simulink model "SPI_controller"  (R2014b)
settings: Solver=FixedStepDiscrete  StartTime=0.0  StopTime=100000  FixedStep=1  RelTol=1e-3
model workspace (MAT data in the model file):
  message_length = Simulink.Parameter
  message_length.Value = 16
  message_length.DataType = 'uint16'
  clk_freq = Simulink.Parameter
  clk_freq.Value = 1000000
  clk_freq.DataType = 'uint32'
  cs_to_clk_edge = Simulink.Parameter
  cs_to_clk_edge.Value = 10
  cs_to_clk_edge.DataType = 'uint16'
  stall_time = Simulink.Parameter
  stall_time.Value = 4
  stall_time.DataType = 'uint16'
undefined symbols (not defined in the file): read_table
libraries: simulink x9, hdlsllib x1
settings Model: FPTRunName=FPA_Reference  Creator=bsoheili  LastModifiedBy=dlwalter
settings DataIOCC: SaveOutput=off  SaveTime=off
settings OptimizationCC: BlockReduction=off  ConditionallyExecuteInputs=off  InlineParams=on  UseDivisionForNetSlopeComputation=UseDivisionForReciprocalsOfIntegersOnly  UseFloatMulNetSlope=on  InlineInvariantSignals=on  EnhancedBackFolding=on  EfficientFloat2IntCast=on  OptimizeModelRefInitCode=on  LifeSpan=1  SimCompilerOptimization=off
settings DebuggingCC: SignalRangeChecking=warning  AlgebraicLoopMsg=error  InheritedTsInSrcMsg=none  ParameterDowncastMsg=warning  ParameterOverflowMsg=warning  FrameProcessingCompatibilityMsg=error  StrictBusMsg=ErrorOnBusTreatedAsVector  NonBusSignalsTreatedAsBus=error
settings HardwareCC: ProdHWDeviceType=ASIC/FPGA->ASIC/FPGA  ProdEqTarget=off
settings RTWCC: SystemTargetFile=ert.tlc  TemplateMakefile=ert_default_tmf  Description=Embedded Coder  GenerateReport=on  IncludeHyperlinkInReport=on  LaunchReport=on  GenerateTraceInfo=on  GenerateTraceReport=on  GenerateTraceReportSl=on  GenerateTraceReportSf=on  GenerateTraceReportEml=on  GenerateCodeMetricsReport=on  RTWCompilerOptimization=off
settings CodeAppCC: IgnoreCustomStorageClasses=off
settings ERTTargetCC: GenerateSampleERTMain=on  CombineSignalStateStructs=on  SuppressErrorStatus=on  InlinedParameterPlacement=NonHierarchical  ERTCustomFileTemplate=example_file_process.tlc

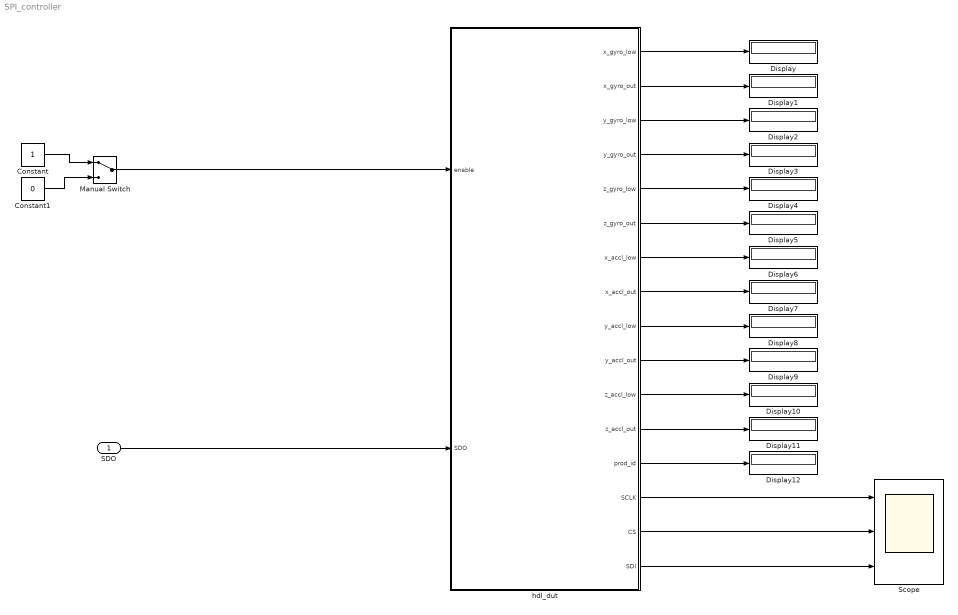
== system SPI_controller ==
  SDO : Inport
  Constant : Constant  OutDataTypeStr=boolean  SampleTime=-1
  Constant1 : Constant  Value=0  OutDataTypeStr=boolean  SampleTime=-1
  Display{,1..12} (13 alike) : Display
  Manual Switch : ManualSwitch
  Scope : Scope  NumInputPorts=3
      settings: TimeRange=3000  YMin=-5~-5~-5  YMax=5~5~5
  hdl_dut : Subsystem  TreatAsAtomicUnit=on  MinMaxOverflowLogging=MinMaxAndOverflow
  wires:
  Manual Switch/1 -> hdl_dut/1(enable)
  SDO/1 -> hdl_dut/2(SDO)
  hdl_dut/1(x_gyro_low) -> Display/1
  hdl_dut/2(x_gyro_out) -> Display1/1
  hdl_dut/3(y_gyro_low) -> Display2/1
  hdl_dut/4(y_gyro_out) -> Display3/1
  hdl_dut/6(z_gyro_out) -> Display5/1
  hdl_dut/5(z_gyro_low) -> Display4/1
  hdl_dut/7(x_accl_low) -> Display6/1
  hdl_dut/8(x_accl_out) -> Display7/1
  hdl_dut/9(y_accl_low) -> Display8/1
  hdl_dut/10(y_accl_out) -> Display9/1
  hdl_dut/11(z_accl_low) -> Display10/1
  hdl_dut/12(z_accl_out) -> Display11/1
  hdl_dut/13(prod_id) -> Display12/1
  hdl_dut/14(SCLK) -> Scope/1
  hdl_dut/15(CS) -> Scope/2
  hdl_dut/16(SDI) -> Scope/3
  Constant/1 -> Manual Switch/1
  Constant1/1 -> Manual Switch/2

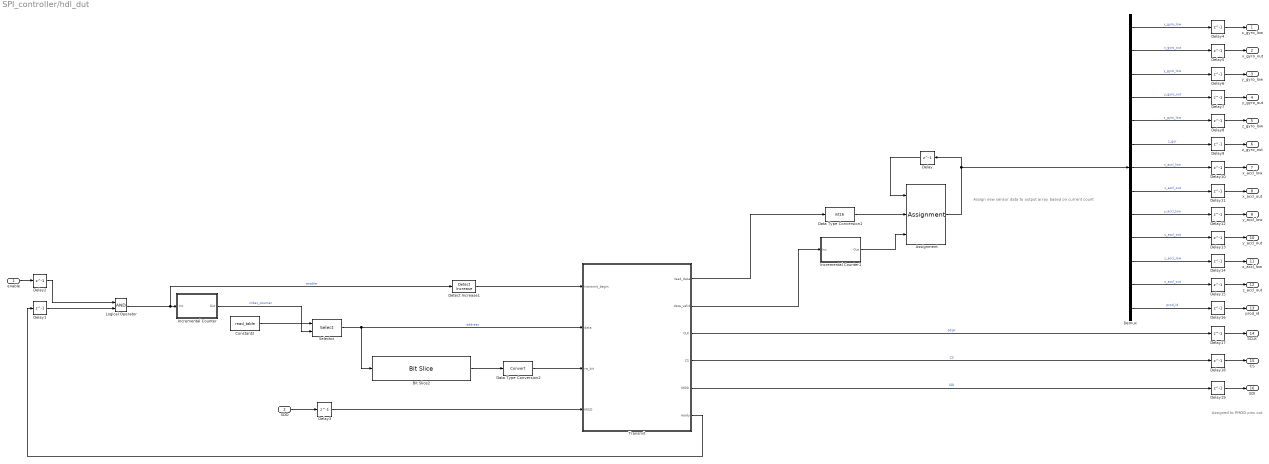
== system SPI_controller/hdl_dut ==
  note: Assign new sensor data to output array based on current count
  note: Assigned to PMOD pins out
  enable : Inport
  SDO : Inport  Port=2
  Assignment : Assignment  DiagnosticForDimensions=Warning  IndexOptions=Index vector (port)  OutputSizes=size(read_table,2)
  Bit Slice2 : hdlsllib/HDL Operations/Bit Slice  lidx=message_length-1  ridx=message_length-1
  Constant2 : Constant  Value=read_table  OutDataTypeStr=uint16  SampleTime=-1
  Data Type Conversion1 : DataTypeConversion  OutDataTypeStr=int16  ConvertRealWorld=Stored Integer (SI)
  Data Type Conversion2 : DataTypeConversion
  Delay : Delay  DelayLength=1  InitialCondition=zeros(1,size(read_table,2))
  Delay1 : Delay  DelayLength=1  InitialCondition=1
  Delay{4..19} (16 alike) : Delay  DelayLength=1  InitialCondition=0
  Delay2 : Delay  DelayLength=1  InitialCondition=1
  Delay3 : Delay  DelayLength=1  InitialCondition=1
  Demux : Demux  Outputs=13
  Detect Increase1 : simulink/Logic and Bit Operations/Detect Increase  vinit=0  InputProcessing=Inherited  OutDataTypeStr=boolean
  Incremental Counter : Subsystem
  Incremental Counter1 : Subsystem
  Logical Operator : Logic  AllPortsSameDT=off  OutDataTypeStr=boolean
  Selector : Selector  InputPortWidth=size(read_table,2)  IndexOptions=Index vector (port)  Indices=[1 3]
  Transmit : Stateflow chart  TreatAsAtomicUnit=on
  x_gyro_low : Outport
  x_gyro_out : Outport  Port=2
  y_gyro_low : Outport  Port=3
  y_gyro_out : Outport  Port=4
  z_gyro_low : Outport  Port=5
  z_gyro_out : Outport  Port=6
  x_accl_low : Outport  Port=7
  x_accl_out : Outport  Port=8
  y_accl_low : Outport  Port=9
  y_accl_out : Outport  Port=10
  z_accl_low : Outport  Port=11
  z_accl_out : Outport  Port=12
  prod_id : Outport  Port=13
  SCLK : Outport  Port=14
  CS : Outport  Port=15
  SDI : Outport  Port=16
  wires:
  Transmit/3(CLK) -> Delay17/1  "SCLK"
  Transmit/4(CS) -> Delay18/1  "CS"
  Transmit/5(MOSI) -> Delay19/1  "SDI"
  Demux/9 -> Delay12/1  "y_accl_low"
  Demux/13 -> Delay16/1  "prod_id"
  Demux/11 -> Delay14/1  "z_accl_low"
  Assignment/1 -> Delay/1, Demux/1
  Demux/12 -> Delay15/1  "z_accl_out"
  Demux/10 -> Delay13/1  "y_accl_out"
  enable/1 -> Delay2/1
  Constant2/1 -> Selector/1
  Transmit/6(ready) -> Delay1/1
  SDO/1 -> Delay3/1
  Delay1/1 -> Logical Operator/2
  Incremental Counter/1(Out) -> Selector/2  "index_counter"
  Delay/1 -> Assignment/1
  Delay2/1 -> Logical Operator/1
  Delay4/1 -> x_gyro_low/1
  Delay5/1 -> x_gyro_out/1
  Delay6/1 -> y_gyro_low/1
  Delay7/1 -> y_gyro_out/1
  Delay8/1 -> z_gyro_low/1
  Delay9/1 -> z_gyro_out/1
  Delay10/1 -> x_accl_low/1
  Delay11/1 -> x_accl_out/1
  Delay13/1 -> y_accl_out/1
  Delay14/1 -> z_accl_low/1
  Delay15/1 -> z_accl_out/1
  Delay16/1 -> prod_id/1
  Delay17/1 -> SCLK/1
  Delay18/1 -> CS/1
  Delay19/1 -> SDI/1
  Detect Increase1/1 -> Transmit/1(transmit_begin)
  Logical Operator/1 -> Incremental Counter/1(Inc), Detect Increase1/1  "enable"
  Delay3/1 -> Transmit/4(MISO)
  Data Type Conversion2/1 -> Transmit/3(rw_bit)
  Selector/1 -> Transmit/2(data), Bit Slice2/1  "address"
  Bit Slice2/1 -> Data Type Conversion2/1
  Demux/1 -> Delay4/1  "x_gyro_low"
  Delay12/1 -> y_accl_low/1
  Demux/2 -> Delay5/1  "x_gyro_out"
  Demux/3 -> Delay6/1  "y_gyro_low"
  Demux/4 -> Delay7/1  "y_gyro_out"
  Demux/5 -> Delay8/1  "z_gyro_low"
  Demux/6 -> Delay9/1  "z_gyr"
  Demux/7 -> Delay10/1  "x_accl_low"
  Demux/8 -> Delay11/1  "x_accl_out"
  Transmit/1(read_data) -> Data Type Conversion1/1
  Data Type Conversion1/1 -> Assignment/2
  Incremental Counter1/1(Out) -> Assignment/3
  Transmit/2(data_valid) -> Incremental Counter1/1(Inc)

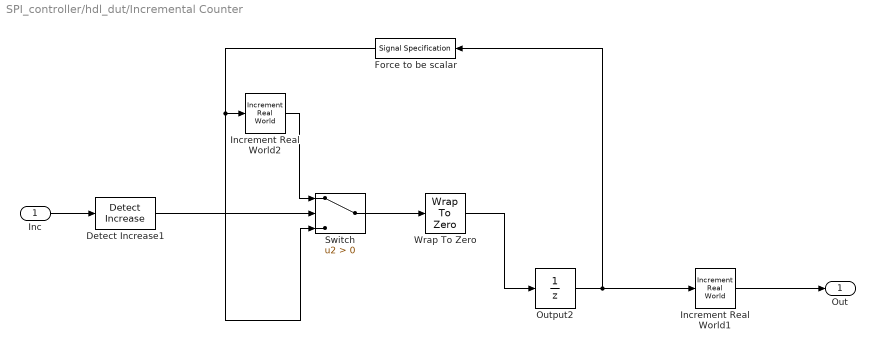
== system SPI_controller/hdl_dut/Incremental Counter ==
  Inc : Inport
  Detect Increase1 : simulink/Logic and Bit Operations/Detect Increase  vinit=0  InputProcessing=Inherited  OutDataTypeStr=boolean
  Force to be scalar : SignalSpecification  DisableCoverage=on  OutDataTypeStr=uint16  Dimensions=1
  Increment Real World1 : simulink/Additional Math & Discrete/Additional Math: Increment - Decrement/Increment Real World  DisableCoverage=on
  Increment Real World2 : simulink/Additional Math & Discrete/Additional Math: Increment - Decrement/Increment Real World  DisableCoverage=on
  Output2 : UnitDelay  SampleTime=-1
  Switch : Switch  Criteria=u2 > Threshold
  Wrap To Zero : simulink/Discontinuities/Wrap To Zero  DisableCoverage=on  Threshold=size(read_table,2)-1
  Out : Outport  InitialOutput=0
  wires:
  Wrap To Zero/1 -> Output2/1
  Switch/1 -> Wrap To Zero/1
  Inc/1 -> Detect Increase1/1
  Force to be scalar/1 -> Switch/3, Increment Real World2/1
  Output2/1 -> Increment Real World1/1, Force to be scalar/1
  Increment Real World2/1 -> Switch/1
  Detect Increase1/1 -> Switch/2
  Increment Real World1/1 -> Out/1

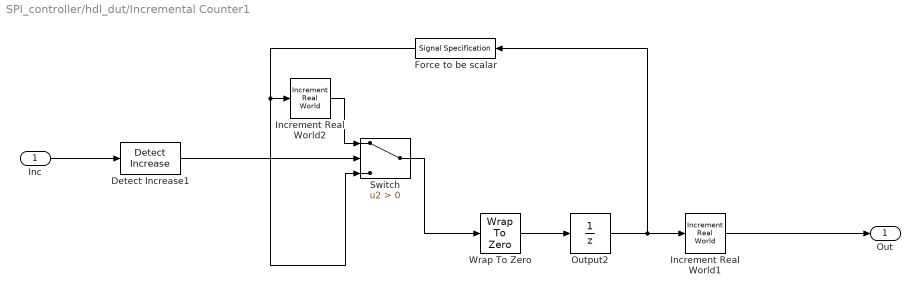
== system SPI_controller/hdl_dut/Incremental Counter1 ==
  Inc : Inport
  Detect Increase1 : simulink/Logic and Bit Operations/Detect Increase  vinit=0  InputProcessing=Inherited  OutDataTypeStr=boolean
  Force to be scalar : SignalSpecification  DisableCoverage=on  OutDataTypeStr=uint16  Dimensions=1
  Increment Real World1 : simulink/Additional Math & Discrete/Additional Math: Increment - Decrement/Increment Real World  DisableCoverage=on
  Increment Real World2 : simulink/Additional Math & Discrete/Additional Math: Increment - Decrement/Increment Real World  DisableCoverage=on
  Output2 : UnitDelay  SampleTime=-1
  Switch : Switch  Criteria=u2 > Threshold
  Wrap To Zero : simulink/Discontinuities/Wrap To Zero  DisableCoverage=on  Threshold=size(read_table,2)-1
  Out : Outport  InitialOutput=0
  wires:
  Increment Real World2/1 -> Switch/1
  Increment Real World1/1 -> Out/1
  Output2/1 -> Increment Real World1/1, Force to be scalar/1
  Force to be scalar/1 -> Increment Real World2/1, Switch/3
  Inc/1 -> Detect Increase1/1
  Switch/1 -> Wrap To Zero/1
  Wrap To Zero/1 -> Output2/1
  Detect Increase1/1 -> Switch/2

== stateflow chart SPI_controller/hdl_dut/Transmit ==
  settings: executeAtInitialization=1
  state IDLE
  state BEGIN
  state CHIPSELECT
  state WRITE
    state CLOCK_BEGIN
    state CLOCK_HIGH
    state CLOCK_LOW
    state CLOCK_END
    (default) -> CLOCK_BEGIN
    CLOCK_BEGIN -> CLOCK_LOW : {CLK = false;
        | bit_count = 0;
        | MOSI = sdi_gen(data,1);}
    CLOCK_LOW -> CLOCK_HIGH [order 1] : [count == clk_wait]
        | {CLK = 1; count = 0;bit_count ++;}
    CLOCK_HIGH -> CLOCK_HIGH [order 3] : {count++;}
    CLOCK_LOW -> CLOCK_LOW [order 2] : {count++;}
    CLOCK_HIGH -> CLOCK_LOW [order 1] : [count == clk_wait]
        | {CLK = 0; count = 0;
        | MOSI = sdi_gen(data, bit_count+1);}
    CLOCK_HIGH -> CLOCK_END [order 2] : [bit_count == message_length]
        | {count = 0; transmit_flag = 0; MOSI = 0;}
  state READ
    state CLOCK_BEGIN1
    state BEGIN_READ
    state CLOCK_HIGH1
    state CLOCK_LOW1
    state CS_LOW
    state CLOCK_BEGIN2
    state CLOCK_END1
    state STALL1
    state CLOCK_HIGH2
    state CLOCK_LOW2
    state DATA_VALID
    state CLK_END
    (default) -> CLOCK_BEGIN1
    CLOCK_BEGIN1 -> CLOCK_LOW1 : {CLK = false;
        | bit_count = 0;
        | MOSI = sdi_gen(data, 1);}
    STALL1 -> BEGIN_READ [order 1] : [count == stall_wait]
        | {count = 0;}
    BEGIN_READ -> BEGIN_READ [order 2] : {count++;}
    CLOCK_LOW1 -> CLOCK_HIGH1 [order 1] : [count == clk_wait]
        | {CLK = 1; count = 0;bit_count ++;}
    CLOCK_HIGH1 -> CLOCK_HIGH1 [order 3] : {count++;}
    CLOCK_LOW1 -> CLOCK_LOW1 [order 2] : {count++;}
    BEGIN_READ -> CS_LOW [order 1] : [count == 10]{CS = 0;count = 0;}
    CLOCK_HIGH1 -> CLOCK_LOW1 [order 1] : [count == clk_wait]
        | {CLK = 0; count = 0;
        | MOSI = sdi_gen(data, bit_count+1);}
    CLOCK_HIGH1 -> CLOCK_END1 [order 2] : [bit_count == message_length]
        | {count = 0; MOSI = 0;}
    CS_LOW -> CS_LOW [order 2] : {count++;}
    CS_LOW -> CLOCK_BEGIN2 [order 1] : [count == cs_wait]
        | {count = 0;}
    CLOCK_END1 -> CLOCK_END1 [order 2] : {count++;}
    STALL1 -> STALL1 [order 2] : {count++;}
    CLOCK_END1 -> STALL1 [order 1] : [count == cs_wait]
        | {count = 0; CS = 1;}
    CLOCK_BEGIN2 -> CLOCK_LOW2 : {CLK = false;
        | bit_count = 0;  read_temp = 0;}
    CLOCK_LOW2 -> CLOCK_HIGH2 [order 1] : [count == clk_wait]
        | {CLK = 1; count = 0;bit_count ++;
        | read_bit = int16(MISO);
        | read_temp = read_temp<<1;
        | read_temp = read_temp|read_bit;}
    CLOCK_HIGH2 -> CLOCK_HIGH2 [order 3] : {count++;}
    CLOCK_LOW2 -> CLOCK_LOW2 [order 2] : {count++;}
    CLOCK_HIGH2 -> CLOCK_LOW2 [order 1] : [count == clk_wait]
        | {CLK = 0; count = 0;}
    CLOCK_HIGH2 -> DATA_VALID [order 2] : [bit_count == message_length]
        | {count = 0; MOSI = 0; data_valid = 1; }
    DATA_VALID -> CLK_END : {read_data= read_temp; transmit_flag = 0;}
  state END_TRANS
  state STALL
  (default) -> IDLE
  STALL -> IDLE [order 1] : [count == stall_wait]
      | {ready = 1;}
  IDLE -> BEGIN : [transmit_begin == 1]
      | {ready = 0;transmit_flag = 1;count = 0;CS = 1; CLK = 1;}
  BEGIN -> CHIPSELECT : {CS = 0;}
  CHIPSELECT -> CHIPSELECT [order 2] : {count++;}
  CHIPSELECT -> (junction 228) [order 1] : [count == cs_wait]{count = 0;}
  (junction 228) -> READ [order 1] : [rw_bit == 0]
  (junction 228) -> WRITE [order 2] : [rw_bit == 1]
  WRITE -> END_TRANS : [transmit_flag == 0]
  READ -> END_TRANS : [transmit_flag == 0]
      | {data_valid = 0;}
  END_TRANS -> END_TRANS [order 2] : {count++;}
  END_TRANS -> STALL [order 1] : [count == cs_wait]{count = 0; CS = 1;}
  STALL -> STALL [order 2] : {count++;}
  data: address function_input uint16; dummy_y function_output uint16; word function_input fixdt(0,16,0); cnt function_input fixdt(0,5,0); ser_data function_output boolean; read_data output uint16; data_valid output boolean =0; CLK output boolean =true; CS output boolean =true; MOSI output boolean; clk_wait local fixdt(0,16,0) =floor(12.5e6/clk_freq); stall_wait local fixdt(0,16,0) =ceil(stall_time/.04); cs_wait local fixdt(0,16,0) =ceil(cs_to_clk_edge/40); count local fixdt(0,16,0); bit_count local fixdt(0,16,0); transmit_flag local boolean; read_bit local uint16; read_temp local uint16; transmit_begin input boolean; data input fixdt(0,message_length,0); rw_bit input boolean; MISO input boolean; clk_freq constant fixdt(0,32,0) =1e6; stall_time constant fixdt(0,16,0) =4; cs_to_clk_edge constant fixdt(0,32,0) =10; message_length constant fixdt(0,16,0) =8; ready output boolean =1
  function dummy_y = dummy_func(address):
    | function dummy_y = dummy_func(address)
    | 
    | 
    | if address == 4096
    |         dummy_out = uint16(1);
    | elseif address == 4608
    |         dummy_out = uint16(2);
    | elseif address == 5120
    |         dummy_out = uint16(3);
    | elseif address == 5632
    |         dummy_out = uint16(4);        
    | elseif address == 6144
    |         dummy_out = uint16(5);
    | elseif address == 6656
    |         dummy_out = uint16(6);
    | elseif address == 7168
    |         dummy_out = uint16(7);
    | elseif address == 7680
    |         dummy_out = uint16(8);
    | elseif address == 8192
    |         dummy_out = uint16(9);
    | elseif address == 8704
    |         dummy_out = uint16(10);
    | elseif address == 9216
    |         dummy_out = uint16(11);        
    | elseif address == 9728
    |         dummy_out = uint16(12);   
    | elseif address == 32256
    |         dummy_out = uint16(16488);  
    | else 
    |     dummy_out = uint16(0);
    | end
    |     
    | dummy_y = dummy_out;
  function ser_data = sdi_gen(word,cnt):
    | function ser_data = sdi_gen(word,cnt)
    | 
    | 
    | persistent ser_data_int;
    | if isempty(ser_data_int)
    |     ser_data_int = false;
    | end
    | 
    | 
    | if cnt == fi(1,0,5,0)
    |     ser_data_int = logical(bitget(word, 16));
    | elseif cnt == fi(2,0,5,0)
    |     ser_data_int = logical(bitget(word, 15));
    | elseif cnt == fi(3,0,5,0)
    |     ser_data_int = logical(bitget(word, 14));
    | elseif cnt == fi(4,0,5,0)
    |     ser_data_int = logical(bitget(word, 13));
    | elseif cnt == fi(5,0,5,0)
    |     ser_data_int = logical(bitget(word, 12));
    | elseif cnt == fi(6,0,5,0)
    |     ser_data_int = logical(bitget(word, 11));
    | elseif cnt == fi(7,0,5,0)
    |     ser_data_int = logical(bitget(word, 10));
    | elseif cnt == fi(8,0,5,0)
    |     ser_data_int = logical(bitget(word, 9));
    | elseif cnt == fi(9,0,5,0)
    |     ser_data_int = logical(bitget(word, 8));
    | elseif cnt == fi(10,0,5,0)
    |     ser_data_int = logical(bitget(word, 7));
    | elseif cnt == fi(11,0,5,0)
    |     ser_data_int = logical(bitget(word, 6));
    | elseif cnt == fi(12,0,5,0)
    |     ser_data_int = logical(bitget(word, 5));
    | elseif cnt == fi(13,0,5,0)
    |     ser_data_int = logical(bitget(word, 4));
    | elseif cnt == fi(14,0,5,0)
    |     ser_data_int = logical(bitget(word, 3));
    | elseif cnt == fi(15,0,5,0)
    |     ser_data_int = logical(bitget(word, 2));
    | elseif cnt == fi(16,0,5,0)
    |     ser_data_int = logical(bitget(word, 1));    
    | else
    |     ser_data_int = true;
    | end
    | 
    | ser_data = ser_data_int;
